simulink model "HW4_1c_least_squares"  (R2023b)
settings: Solver=VariableStepAuto  StartTime=0.0  StopTime=1000  RelTol=1e-3
model workspace (MAT data in the model file):
  alpha = Simulink.Parameter
  alpha.Value = 1
  alpha.DataType = 'auto'
  alpha.Complexity = 'real'
  alpha.Dimensions = [1 1]
  b = Simulink.Parameter
  b.Value = 0.1
  b.DataType = 'auto'
  b.Complexity = 'real'
  b.Dimensions = [1 1]
  beta = Simulink.Parameter
  beta.Value = 1
  beta.DataType = 'auto'
  beta.Complexity = 'real'
  beta.Dimensions = [1 1]
  k = Simulink.Parameter
  k.Value = 5
  k.DataType = 'auto'
  k.Complexity = 'real'
  k.Dimensions = [1 1]
  m = Simulink.Parameter
  m.Value = 20
  m.DataType = 'auto'
  m.Complexity = 'real'
  m.Dimensions = [1 1]
  minv = Simulink.Parameter
  minv.Value = 0.05
  minv.DataType = 'auto'
  minv.Complexity = 'real'
  minv.Dimensions = [1 1]
libraries: matrix_library x3
settings Model: Creator=kaleb  LastModifiedBy=kaleb

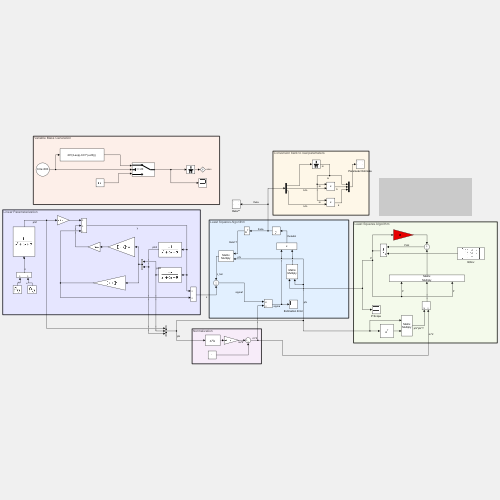
[thumbnail: Simulink's stored preview of the top-level diagram]
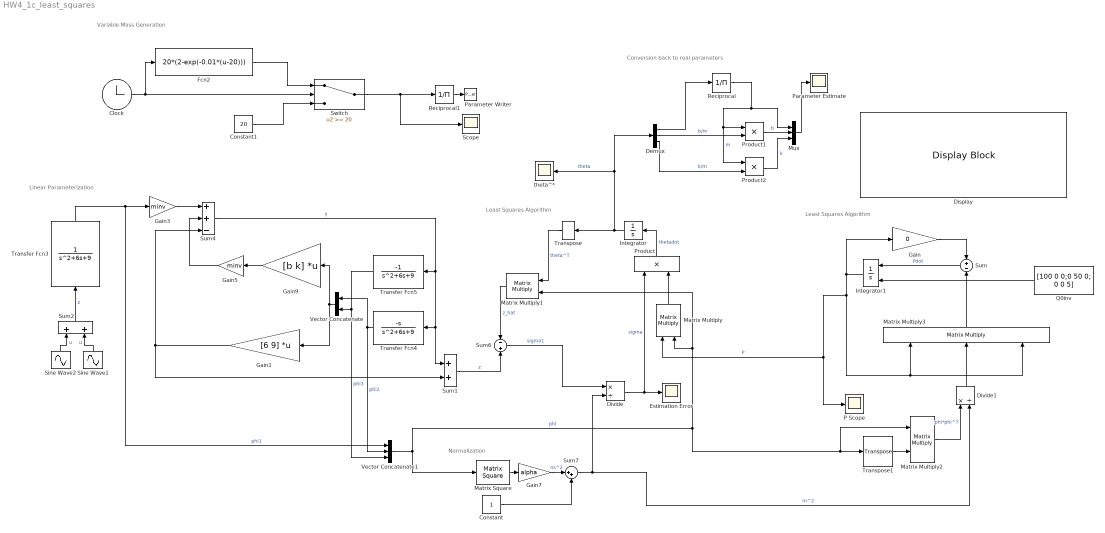
== system HW4_1c_least_squares ==
  note: Variable Mass Generation
  note: Least Squares Algorithm
  note: Least Squares Algorithm
  note: Conversion back to real parameters
  note: Normalization
  note: Linear Parameterization
  Clock : Clock
  Constant : Constant
  Constant1 : Constant  Value=20
  Demux : Demux  Outputs=3
  Display : DisplayBlock  LabelPosition=Hide  Transparency=1
  Divide : Product  Inputs=*/
  Divide1 : Product  Inputs=*/
  Estimation Error : Scope
  Fcn2 : Fcn  Expr=20*(2-exp(-0.01*(u-20)))
  Gain : Gain  Gain=0
  Gain1 : Gain  Gain=[6 9]  Multiplication=Matrix(K*u)
  Gain3 : Gain  Gain=minv
  Gain5 : Gain  Gain=minv
  Gain7 : Gain  Gain=alpha
  Gain9 : Gain  Gain=[b k]  Multiplication=Matrix(K*u)
  Integrator : Integrator  InitialCondition=[0.1 0.15 0.3]
  Integrator1 : Integrator  InitialConditionSource=external  InitialCondition=[1 0 0; 0 1 0; 0 0 1]
  Matrix Square : matrix_library/Matrix Square  OutMin=[]  OutMax=[]
      settings: LibrarySourceBlock=|
      | simulink/Matrix
      | Operations/Matrix
      | Square
  Matrix Multiply : Product  Multiplication=Matrix(*)
  Matrix Multiply1 : Product  Multiplication=Matrix(*)
  Matrix Multiply2 : Product  Multiplication=Matrix(*)
  Matrix Multiply3 : Product  Inputs=3  Multiplication=Matrix(*)
  Mux : Mux  Inputs=3
  P Scope : Scope
  Parameter Estimate : Scope
  Parameter Writer : ParameterWriter  AccessWorkspaceVariable=on  WorkspaceVariableName=minv
  Product : Product
  Product1 : Product
  Product2 : Product
  Q0inv : Constant  Value=[100 0 0;0 50 0; 0 0 5]
  Reciprocal : Product  Inputs=/  OutMax=[10000]
  Reciprocal1 : Product  Inputs=/
  Scope : Scope
  Sine Wave1 : Sin  Amplitude=5  Frequency=3  SampleTime=0
  Sine Wave2 : Sin  Amplitude=3  Frequency=1.5  SampleTime=0
  Sum : Sum  Inputs=+-
  Sum1 : Sum
  Sum2 : Sum
  Sum4 : Sum  Inputs=++-
  Sum6 : Sum  Inputs=-+
  Sum7 : Sum  Inputs=|++
  Switch : Switch  Threshold=20  ZeroCross=off  SaturateOnIntegerOverflow=off  InputSameDT=off
  Transfer Fcn3 : TransferFcn  Denominator=[1 6 9]
  Transfer Fcn4 : TransferFcn  Numerator=[-1 0]  Denominator=[1 6 9]
  Transfer Fcn5 : TransferFcn  Numerator=[-1]  Denominator=[1 6 9]
  Transpose : matrix_library/Transpose
  Transpose1 : matrix_library/Transpose
  Vector Concatenate : Concatenate
  Vector Concatenate1 : Concatenate  NumInputs=3
  theta^* : Scope
  wires:
  Sine Wave1/1 -> Sum2/2  "u"
  Transfer Fcn3/1 -> Vector Concatenate1/1, Gain3/1  "phi1"
  Sum4/1 -> Transfer Fcn5/1, Sum1/1, Transfer Fcn4/1  "y"
  Transfer Fcn4/1 -> Vector Concatenate/1, Vector Concatenate1/2  "phi2"
  Transfer Fcn5/1 -> Vector Concatenate/2, Vector Concatenate1/3  "phi3"
  Gain9/1 -> Gain5/1
  Vector Concatenate1/1 -> Matrix Multiply2/1, Transpose1/1, Matrix Multiply1/2, Matrix Multiply/2, Matrix Square/1  "phi"
  Matrix Multiply1/1 -> Sum6/1  "z_hat"
  Matrix Square/1 -> Gain7/1
  Constant/1 -> Sum7/2
  Sum7/1 -> Divide1/2, Divide/2  "m^2"
  Gain7/1 -> Sum7/1  "ns^2"
  Sum6/1 -> Divide/1  "sigma1"
  Product/1 -> Integrator/1  "thetadot"
  Integrator/1 -> Transpose/1, Demux/1, theta^*/1  "theta"
  Transpose/1 -> Matrix Multiply1/1  "theta^T"
  Divide/1 -> Estimation Error/1, Product/1  "sigma"
  Demux/2 -> Product1/2  "b/m"
  Demux/3 -> Product2/2  "k/m"
  Reciprocal/1 -> Product1/1, Product2/1, Mux/1  "m"
  Product1/1 -> Mux/2  "b"
  Product2/1 -> Mux/3  "k"
  Mux/1 -> Parameter Estimate/1
  Matrix Multiply/1 -> Product/2
  Demux/1 -> Reciprocal/1
  Vector Concatenate/1 -> Gain9/1, Gain1/1
  Gain1/1 -> Sum4/3, Sum1/2
  Sum1/1 -> Sum6/2  "z"
  Sum/1 -> Integrator1/1  "Pdot"
  Integrator1/1 -> Gain/1, Matrix Multiply/1, P Scope/1, Matrix Multiply3/3, Matrix Multiply3/1  "P"
  Gain/1 -> Sum/1
  Transpose1/1 -> Matrix Multiply2/2
  Matrix Multiply2/1 -> Divide1/1  "phi*phi^T"
  Matrix Multiply3/1 -> Sum/2
  Divide1/1 -> Matrix Multiply3/2
  Q0inv/1 -> Integrator1/2
  Sine Wave2/1 -> Sum2/1  "u"
  Sum2/1 -> Transfer Fcn3/1  "z"
  Clock/1 -> Fcn2/1, Switch/2
  Fcn2/1 -> Switch/1
  Gain3/1 -> Sum4/1
  Gain5/1 -> Sum4/2
  Reciprocal1/1 -> Parameter Writer/1
  Constant1/1 -> Switch/3
  Switch/1 -> Scope/1, Reciprocal1/1
